simulink model "GVCU_HIL_simscape"  (R2026a)
settings: Solver=ode3  StartTime=0  StopTime=10  FixedStep=0.001
model workspace (MAT data in the model file):
  CANoelibParameters : object (value not decoded)
values from neighbouring files (symbols this model uses):
  acc_pedal_data = pedal_data.accelerator_pedal_position_t0    [Init_Simscape_main.m]
  acc_pedal_time = pedal_data.t0    [Init_Simscape_main.m]
  brk_pedal_data = brake_pedal_data.shared_brakes_drvrBrkPedlPerc_t0    [Init_Simscape_main.m]
  brk_pedal_time = brake_pedal_data.t0    [Init_Simscape_main.m]
  cycle_len = zeros(1, num_cycles)    [Init_Simscape_main.m]
  cycle_speed_matrix = zeros(max_cycle_len, num_cycles)    [Init_Simscape_main.m]
  cycle_time_matrix = zeros(max_cycle_len, num_cycles)    [Init_Simscape_main.m]
  veh_speed_data = speed_data.shared_dynamicsVso_vehVelLgt_t0    [Init_Simscape_main.m]
  veh_speed_time = speed_data.t0    [Init_Simscape_main.m]
undefined symbols (not defined in the file or in its folder): Active, aero, AuxActive, bat, brake, config, environment, FL, FL_prs_voltage, FR, FR_prs_voltage, front, pos, powertrain, rear, RL, RL_prs_voltage, RR, RR_prs_voltage, tir, veh, VGetRawValueFlag, Voltage, VT2816_1_Ch1, VT2816_1_Ch2, VT2816_1_Ch3, VT2816_1_Ch4, VT2816_3_Ch13, VT2816_3_Ch14, VT7101_1_Out2, VTS, X, Y, Z
libraries: sm_lib x358, fl_lib x272, nesl_utility x193, canoelib x127, sdl_lib x36, autolibsharedcoupling x21, autolibcoupling x9, slpidlib x7, simulink x3, autolibshareddiff x3, autolibshared x3, autolibutils x1
(part 4 of 17)

== system GVCU_HIL_simscape/GVCU - HiL/Message Output17 ==
  In1 : Inport
  Bus Selector : BusSelector  OutputSignals=available_charge_current,available_discharge_current,bms_state,dcdc_contactor,e2e_alive_counter_disabled,e2e_checksum_disabled,front_hv_bat_fan_req,front_hv_bat_pump_req,hv_on_req_lv_charging,hvac_contactor,obc_contactor
  S-Function_1 : S-Function  FunctionName=sigout  Parameters=dbName;nodeName;msgName;11;'available_charge_current';'available_discharge_current';'bms_state';'dcdc_contactor';'e2e_alive_counter_disabled';'e2e_checksum_disabled';'front_hv_bat_fan_req';'front_hv_bat_pump_req';'hv_on_req_lv_charging';'hvac_contactor';'obc_contactor';VGetRawValueFlag(rawValue);'inherited'  SFunctionDeploymentMode=off  EnableBusSupport=off
      settings: AttributesFormatString=available_charge_current\navailable_discharge_current\nbms_state\ndcdc_contactor\ne2e_alive_counter_disabled\ne2e_checksum_disabled\nfront_hv_bat_fan_req\nfront_hv_bat_pump_req\nhv_on_req_lv_charging\nhvac_contactor\nobc_contactor\n
  wires:
  In1/1 -> Bus Selector/1
  Bus Selector/1 -> S-Function_1/1  "<available_charge_current>"
  Bus Selector/2 -> S-Function_1/2  "<available_discharge_current>"
  Bus Selector/3 -> S-Function_1/3  "<bms_state>"
  Bus Selector/4 -> S-Function_1/4  "<dcdc_contactor>"
  Bus Selector/5 -> S-Function_1/5  "<e2e_alive_counter_disabled>"
  Bus Selector/6 -> S-Function_1/6  "<e2e_checksum_disabled>"
  Bus Selector/7 -> S-Function_1/7  "<front_hv_bat_fan_req>"
  Bus Selector/8 -> S-Function_1/8  "<front_hv_bat_pump_req>"
  Bus Selector/9 -> S-Function_1/9  "<hv_on_req_lv_charging>"
  Bus Selector/10 -> S-Function_1/10  "<hvac_contactor>"
  Bus Selector/11 -> S-Function_1/11  "<obc_contactor>"

== system GVCU_HIL_simscape/GVCU - HiL/Message Output18 ==
  In1 : Inport
  Bus Selector : BusSelector  OutputSignals=e2e_alive_counter_disabled,e2e_checksum_disabled,soc,soc_predictive,soc_predictive_v,soc_v,soe,soe_v,soh,soh_v,thermal_runaway_detection
  S-Function_1 : S-Function  FunctionName=sigout  Parameters=dbName;nodeName;msgName;11;'e2e_alive_counter_disabled';'e2e_checksum_disabled';'soc';'soc_predictive';'soc_predictive_v';'soc_v';'soe';'soe_v';'soh';'soh_v';'thermal_runaway_detection';VGetRawValueFlag(rawValue);'inherited'  SFunctionDeploymentMode=off  EnableBusSupport=off
      settings: AttributesFormatString=e2e_alive_counter_disabled\ne2e_checksum_disabled\nsoc\nsoc_predictive\nsoc_predictive_v\nsoc_v\nsoe\nsoe_v\nsoh\nsoh_v\nthermal_runaway_detection\n
  wires:
  In1/1 -> Bus Selector/1
  Bus Selector/10 -> S-Function_1/1, S-Function_1/10  "<soh_v>"
  Bus Selector/1 -> S-Function_1/2  "<e2e_alive_counter_disabled>"
  Bus Selector/2 -> S-Function_1/3  "<e2e_checksum_disabled>"
  Bus Selector/3 -> S-Function_1/4  "<soc>"
  Bus Selector/7 -> S-Function_1/5  "<soe>"
  Bus Selector/9 -> S-Function_1/6, S-Function_1/9  "<soh>"
  Bus Selector/11 -> S-Function_1/7, S-Function_1/11  "<thermal_runaway_detection>"
  Bus Selector/8 -> S-Function_1/8  "<soe_v>"

== system GVCU_HIL_simscape/GVCU - HiL/Message Output2 ==
  In1 : Inport
  Bus Selector : BusSelector  OutputSignals=third_shaft_speed,third_shaft_speed_v
  S-Function_1 : S-Function  FunctionName=sigout  Parameters=dbName;nodeName;msgName;2;'third_shaft_speed';'third_shaft_speed_v';VGetRawValueFlag(rawValue);'inherited'  SFunctionDeploymentMode=off  EnableBusSupport=off
      settings: AttributesFormatString=third_shaft_speed\nthird_shaft_speed_v\n
  wires:
  In1/1 -> Bus Selector/1
  Bus Selector/1 -> S-Function_1/1  "<third_shaft_speed>"
  Bus Selector/2 -> S-Function_1/2  "<third_shaft_speed_v>"

== system GVCU_HIL_simscape/GVCU - HiL/Message Output21 ==
  In1 : Inport
  Bus Selector : BusSelector  OutputSignals=active_mode,brake_pedal_applied,brake_pedal_travel_mm,brake_pedal_travel_mm_v,brake_pedal_travel_perc,brake_pedal_travel_perc_v,brake_pedal_travel_sensor_sts,e2e_alive_counter,e2e_checksum,position_motor,position_motor_v
  S-Function_1 : S-Function  FunctionName=sigout  Parameters=dbName;nodeName;msgName;11;'active_mode';'brake_pedal_applied';'brake_pedal_travel_mm';'brake_pedal_travel_mm_v';'brake_pedal_travel_perc';'brake_pedal_travel_perc_v';'brake_pedal_travel_sensor_sts';'e2e_alive_counter';'e2e_checksum';'position_motor';'position_motor_v';VGetRawValueFlag(rawValue);'inherited'  SFunctionDeploymentMode=off  EnableBusSupport=off
      settings: AttributesFormatString=active_mode\nbrake_pedal_applied\nbrake_pedal_travel_mm\nbrake_pedal_travel_mm_v\nbrake_pedal_travel_perc\nbrake_pedal_travel_perc_v\nbrake_pedal_travel_sensor_sts\ne2e_alive_counter\ne2e_checksum\nposition_motor\nposition_motor_v\n
  wires:
  In1/1 -> Bus Selector/1
  Bus Selector/7 -> S-Function_1/1  "<brake_pedal_travel_sensor_sts>"
  Bus Selector/1 -> S-Function_1/2  "<active_mode>"
  Bus Selector/4 -> S-Function_1/3  "<brake_pedal_travel_mm_v>"
  Bus Selector/8 -> S-Function_1/4  "<e2e_alive_counter>"
  Bus Selector/9 -> S-Function_1/5  "<e2e_checksum>"
  Bus Selector/11 -> S-Function_1/6, S-Function_1/11  "<position_motor_v>"
  Bus Selector/6 -> S-Function_1/7  "<brake_pedal_travel_perc_v>"
  Bus Selector/2 -> S-Function_1/8  "<brake_pedal_applied>"
  Bus Selector/10 -> S-Function_1/9  "<position_motor>"
  Bus Selector/3 -> S-Function_1/10  "<brake_pedal_travel_mm>"

== system GVCU_HIL_simscape/GVCU - HiL/Message Output3 ==
  In1 : Inport
  Bus Selector : BusSelector  OutputSignals=auto_shift_perf_mod_swt_req,ddc_perf_mod_swt_req,e2e_alive_counter_disabled,e2e_checksum_disabled,eps_perf_mod_swt_req,pedl_map_perf_mod_swt_req,perf_mod_swt_req,perf_stgy_perf_mod_swt_req,rgn_perf_mod_swt_req,rhc_perf_mod_swt_req
  S-Function_1 : S-Function  FunctionName=sigout  Parameters=dbName;nodeName;msgName;10;'auto_shift_perf_mod_swt_req';'ddc_perf_mod_swt_req';'e2e_alive_counter_disabled';'e2e_checksum_disabled';'eps_perf_mod_swt_req';'pedl_map_perf_mod_swt_req';'perf_mod_swt_req';'perf_stgy_perf_mod_swt_req';'rgn_perf_mod_swt_req';'rhc_perf_mod_swt_req';VGetRawValueFlag(rawValue);'inherited'  SFunctionDeploymentMode=off  EnableBusSupport=off
      settings: AttributesFormatString=auto_shift_perf_mod_swt_req\nddc_perf_mod_swt_req\ne2e_alive_counter_disabled\ne2e_checksum_disabled\neps_perf_mod_swt_req\npedl_map_perf_mod_swt_req\nperf_mod_swt_req\nperf_stgy_perf_mod_swt_req\nrgn_perf_mod_swt_req\nrhc_perf_mod_swt_req\n
  wires:
  In1/1 -> Bus Selector/1
  Bus Selector/1 -> S-Function_1/1  "<auto_shift_perf_mod_swt_req>"
  Bus Selector/2 -> S-Function_1/2  "<ddc_perf_mod_swt_req>"
  ? -> S-Function_1/3  "<drift_mod_swt_req>"
  Bus Selector/3 -> S-Function_1/4  "<e2e_alive_counter_disabled>"
  Bus Selector/4 -> S-Function_1/5  "<e2e_checksum_disabled>"
  Bus Selector/5 -> S-Function_1/6  "<eps_perf_mod_swt_req>"
  Bus Selector/6 -> S-Function_1/7  "<pedl_map_perf_mod_swt_req>"
  Bus Selector/7 -> S-Function_1/8  "<perf_mod_swt_req>"
  Bus Selector/8 -> S-Function_1/9  "<perf_stgy_perf_mod_swt_req>"
  Bus Selector/9 -> S-Function_1/10  "<rgn_perf_mod_swt_req>"

== system GVCU_HIL_simscape/GVCU - HiL/Message Output7 ==
  In1 : Inport
  Bus Selector : BusSelector  OutputSignals=dtc_list_12v,dtc_list_48v,e2e_alive_counter_disabled,e2e_checksum_disabled,in_current_hv,in_voltage_hv,state_12v,state_48v,swt_ena_fb_12v,swt_ena_fb_48v
  S-Function_1 : S-Function  FunctionName=sigout  Parameters=dbName;nodeName;msgName;10;'dtc_list_12v';'dtc_list_48v';'e2e_alive_counter_disabled';'e2e_checksum_disabled';'in_current_hv';'in_voltage_hv';'state_12v';'state_48v';'swt_ena_fb_12v';'swt_ena_fb_48v';VGetRawValueFlag(rawValue);'inherited'  SFunctionDeploymentMode=off  EnableBusSupport=off
      settings: AttributesFormatString=dtc_list_12v\ndtc_list_48v\ne2e_alive_counter_disabled\ne2e_checksum_disabled\nin_current_hv\nin_voltage_hv\nstate_12v\nstate_48v\nswt_ena_fb_12v\nswt_ena_fb_48v\n
  wires:
  In1/1 -> Bus Selector/1
  Bus Selector/1 -> S-Function_1/1  "<dtc_list_12v>"
  Bus Selector/2 -> S-Function_1/2  "<dtc_list_48v>"
  Bus Selector/3 -> S-Function_1/3  "<e2e_alive_counter_disabled>"
  Bus Selector/4 -> S-Function_1/4  "<e2e_checksum_disabled>"
  Bus Selector/5 -> S-Function_1/5  "<in_current_hv>"
  Bus Selector/6 -> S-Function_1/6  "<in_voltage_hv>"
  Bus Selector/7 -> S-Function_1/7  "<state_12v>"
  Bus Selector/8 -> S-Function_1/8  "<state_48v>"
  Bus Selector/9 -> S-Function_1/9  "<swt_ena_fb_12v>"
  Bus Selector/10 -> S-Function_1/10  "<swt_ena_fb_48v>"

== system GVCU_HIL_simscape/GVCU - HiL/Message Output8 ==
  In1 : Inport
  Bus Selector : BusSelector  OutputSignals=available_power_12v,available_power_48v,current_output_12v,current_output_48v,dcdc_fan_req,dcdc_pump_req,e2e_alive_counter_disabled,e2e_checksum_disabled
  S-Function_1 : S-Function  FunctionName=sigout  Parameters=dbName;nodeName;msgName;8;'available_power_12v';'available_power_48v';'current_output_12v';'current_output_48v';'dcdc_fan_req';'dcdc_pump_req';'e2e_alive_counter_disabled';'e2e_checksum_disabled';VGetRawValueFlag(rawValue);'inherited'  SFunctionDeploymentMode=off  EnableBusSupport=off
      settings: AttributesFormatString=available_power_12v\navailable_power_48v\ncurrent_output_12v\ncurrent_output_48v\ndcdc_fan_req\ndcdc_pump_req\ne2e_alive_counter_disabled\ne2e_checksum_disabled\n
  wires:
  In1/1 -> Bus Selector/1
  Bus Selector/1 -> S-Function_1/1  "<available_power_12v>"
  Bus Selector/2 -> S-Function_1/2  "<available_power_48v>"
  Bus Selector/3 -> S-Function_1/3  "<current_output_12v>"
  Bus Selector/4 -> S-Function_1/4  "<current_output_48v>"
  Bus Selector/5 -> S-Function_1/5  "<dcdc_fan_req>"
  Bus Selector/6 -> S-Function_1/6  "<dcdc_pump_req>"
  Bus Selector/7 -> S-Function_1/7  "<e2e_alive_counter_disabled>"
  Bus Selector/8 -> S-Function_1/8  "<e2e_checksum_disabled>"

== system GVCU_HIL_simscape/Inverter/Message Output ==
  In1 : Inport
  Bus Selector : BusSelector  OutputSignals=ctrl_mode_feedback,dc_current,dc_voltage,e2e_alive_counter_disabled,e2e_checksum_disabled,fault_level,inv_enable_feedback,motor_enable_feedback,safe_state_method,safe_state_req_feedback,state_machine,torque_limit_reason
  S-Function_1 : S-Function  FunctionName=sigout  Parameters=dbName;nodeName;msgName;12;'ctrl_mode_feedback';'dc_current';'dc_voltage';'e2e_alive_counter_disabled';'e2e_checksum_disabled';'fault_level';'inv_enable_feedback';'motor_enable_feedback';'safe_state_method';'safe_state_req_feedback';'state_machine';'torque_limit_reason';VGetRawValueFlag(rawValue);'inherited'  SFunctionDeploymentMode=off  EnableBusSupport=off
      settings: AttributesFormatString=ctrl_mode_feedback\ndc_current\ndc_voltage\ne2e_alive_counter_disabled\ne2e_checksum_disabled\nfault_level\ninv_enable_feedback\nmotor_enable_feedback\nsafe_state_method\nsafe_state_req_feedback\nstate_machine\ntorque_limit_reason\n
  wires:
  In1/1 -> Bus Selector/1
  Bus Selector/1 -> S-Function_1/1  "<ctrl_mode_feedback>"
  Bus Selector/2 -> S-Function_1/2  "<dc_current>"
  Bus Selector/3 -> S-Function_1/3  "<dc_voltage>"
  Bus Selector/4 -> S-Function_1/4  "<e2e_alive_counter_disabled>"
  Bus Selector/5 -> S-Function_1/5  "<e2e_checksum_disabled>"
  Bus Selector/6 -> S-Function_1/6  "<fault_level>"
  Bus Selector/7 -> S-Function_1/7  "<inv_enable_feedback>"
  Bus Selector/8 -> S-Function_1/8  "<motor_enable_feedback>"
  Bus Selector/9 -> S-Function_1/9  "<safe_state_method>"
  Bus Selector/10 -> S-Function_1/10  "<safe_state_req_feedback>"
  Bus Selector/11 -> S-Function_1/11  "<state_machine>"
  Bus Selector/12 -> S-Function_1/12  "<torque_limit_reason>"

== system GVCU_HIL_simscape/Inverter/Message Output1 ==
  In1 : Inport
  Bus Selector : BusSelector  OutputSignals=e2e_alive_counter_disabled,e2e_checksum_disabled,motor_speed,motor_speed_valid_bit,pos_offset_a,pos_offset_b
  S-Function_1 : S-Function  FunctionName=sigout  Parameters=dbName;nodeName;msgName;6;'e2e_alive_counter_disabled';'e2e_checksum_disabled';'motor_speed';'motor_speed_valid_bit';'pos_offset_a';'pos_offset_b';VGetRawValueFlag(rawValue);'inherited'  SFunctionDeploymentMode=off  EnableBusSupport=off
      settings: AttributesFormatString=e2e_alive_counter_disabled\ne2e_checksum_disabled\nmotor_speed\nmotor_speed_valid_bit\npos_offset_a\npos_offset_b\n
  wires:
  In1/1 -> Bus Selector/1
  Bus Selector/1 -> S-Function_1/1  "<e2e_alive_counter_disabled>"
  Bus Selector/2 -> S-Function_1/2  "<e2e_checksum_disabled>"
  Bus Selector/3 -> S-Function_1/3  "<motor_speed>"
  Bus Selector/4 -> S-Function_1/4  "<motor_speed_valid_bit>"
  Bus Selector/5 -> S-Function_1/5  "<pos_offset_a>"
  Bus Selector/6 -> S-Function_1/6  "<pos_offset_b>"

== system GVCU_HIL_simscape/Inverter/Message Output2 ==
  In1 : Inport
  Bus Selector : BusSelector  OutputSignals=can_comm_loss_error,can_comm_loss_warning,can_e2e,coolant_t_fault,coolant_t_rationality,coolant_t_sensing,coolant_t_warning,crash_signal,dc_link_t_fault,dc_link_t_rationality,dc_link_t_sensing,dc_link_t_warning,driver_t_fault,driver_t_rationality,driver_t_sensing,driver_t_warning,e2e_alive_counter_disabled,e2e_checksum_disabled,gate_driver_bist_fault,gate_driver_fault,gate_driver_warning,inverter_boards_t_fault,inverter_boards_t_rationality,inverter_boards_t_sensing,inverter_boards_t_warning,ipc_lock_cm,ipc_lock_main,lv_ext_supply_ov,lv_ext_supply_uv,lv_int_supply,lv_self_check_main,mcu_bist_fault,mcu_fault,mosfet_t_fault,mosfet_t_imbalance,mosfet_t_rationality,mosfet_t_sensing,mosfet_t_warning,motor_t_fault,motor_t_rationality,motor_t_sensing,motor_t_warning,sbc_bist_fault,sbc_fault,sw_compatibility,task_alive_cm,task_alive_main,task_deadline_cm,task_deadline_main,y_cap_ctrl_u
  S-Function_1 : S-Function  FunctionName=sigout  Parameters=dbName;nodeName;msgName;50;'can_comm_loss_error';'can_comm_loss_warning';'can_e2e';'coolant_t_fault';'coolant_t_rationality';'coolant_t_sensing';'coolant_t_warning';'crash_signal';'dc_link_t_fault';'dc_link_t_rationality';'dc_link_t_sensing';'dc_link_t_warning';'driver_t_fault';'driver_t_rationality';'driver_t_sensing';'driver_t_warning';'e2e_alive_counter_disabled';'e2e_checksum_disabled';'gate_driver_bist_fault';'gate_driver_fault';'gate_driver_warning';'inverter_boards_t_fault';'inverter_boards_t_rationality';'inverter_boards_t_sensing';'inverter_boards_t_warning';'ipc_lock_cm';'ipc_lock_main';'lv_ext_supply_ov';'lv_ext_supply_uv';'lv_int_supply';'lv_self_check_main';'mcu_bist_fault';'mcu_fault';'mosfet_t_fault';'mosfet_t_imbalance';'mosfet_t_rationality';'mosfet_t_sensing';'mosfet_t_warning';'motor_t_fault';'motor_t_rationality';'motor_t_sensing';'motor_t_warning';'sbc_bist_fault';'sbc_fault';'sw_compatibility';'task_alive_cm';'task_alive_main';'task_deadline_cm';'task_deadline_main';'y_cap_ctrl_u';VGetRawValueFlag(rawValue);'inherited'  SFunctionDeploymentMode=off  EnableBusSupport=off
      settings: AttributesFormatString=can_comm_loss_error\ncan_comm_loss_warning\ncan_e2e\ncoolant_t_fault\ncoolant_t_rationality\ncoolant_t_sensing\ncoolant_t_warning\ncrash_signal\ndc_link_t_fault\ndc_link_t_rationality\ndc_link_t_sensing\ndc_link_t_warning\ndriver_t_fault\ndriver_t_rationality\ndriver_t_sensing\ndriver_t_warning\ne2e_alive_counter_disabled\ne2e_checksum_disabled\ngate_driver_bist_fault\ngate_driver_fault\ngate_driver_warning\ninverter_boards_t_fault\ninverter_boards_t_rationality\ninverter_boards_t_sensing\ninverter_boards_t_warning\nipc_lock_cm\nipc_lock_main\nlv_ext_supply_ov\nlv_ext_supply_uv\nlv_int_supply\nlv_self_check_main\nmcu_bist_fault\nmcu_fault\nmosfet_t_fault\nmosfet_t_imbalance\nmosfet_t_rationality\nmosfet_t_sensing\nmosfet_t_warning\nmotor_t_fault\nmotor_t_rationality\nmotor_t_sensing\nmotor_t_warning\nsbc_bist_fault\nsbc_fault\nsw_compatibility\ntask_alive_cm\ntask_alive_main\ntask_deadline_cm\ntask_deadline_main\ny_cap_ctrl_u\n
  wires:
  In1/1 -> Bus Selector/1
  Bus Selector/1 -> S-Function_1/1  "<can_comm_loss_error>"
  Bus Selector/2 -> S-Function_1/2  "<can_comm_loss_warning>"
  Bus Selector/3 -> S-Function_1/3  "<can_e2e>"
  Bus Selector/4 -> S-Function_1/4  "<coolant_t_fault>"
  Bus Selector/5 -> S-Function_1/5  "<coolant_t_rationality>"
  Bus Selector/6 -> S-Function_1/6  "<coolant_t_sensing>"
  Bus Selector/7 -> S-Function_1/7  "<coolant_t_warning>"
  Bus Selector/8 -> S-Function_1/8  "<crash_signal>"
  Bus Selector/9 -> S-Function_1/9  "<dc_link_t_fault>"
  Bus Selector/10 -> S-Function_1/10  "<dc_link_t_rationality>"
  Bus Selector/11 -> S-Function_1/11  "<dc_link_t_sensing>"
  Bus Selector/12 -> S-Function_1/12  "<dc_link_t_warning>"
  Bus Selector/13 -> S-Function_1/13  "<driver_t_fault>"
  Bus Selector/14 -> S-Function_1/14  "<driver_t_rationality>"
  Bus Selector/15 -> S-Function_1/15  "<driver_t_sensing>"
  Bus Selector/16 -> S-Function_1/16  "<driver_t_warning>"
  Bus Selector/17 -> S-Function_1/17  "<e2e_alive_counter_disabled>"
  Bus Selector/18 -> S-Function_1/18  "<e2e_checksum_disabled>"
  Bus Selector/19 -> S-Function_1/19  "<gate_driver_bist_fault>"
  Bus Selector/20 -> S-Function_1/20  "<gate_driver_fault>"
  Bus Selector/21 -> S-Function_1/21  "<gate_driver_warning>"
  Bus Selector/22 -> S-Function_1/22  "<inverter_boards_t_fault>"
  Bus Selector/23 -> S-Function_1/23  "<inverter_boards_t_rationality>"
  Bus Selector/24 -> S-Function_1/24  "<inverter_boards_t_sensing>"
  Bus Selector/25 -> S-Function_1/25  "<inverter_boards_t_warning>"
  Bus Selector/26 -> S-Function_1/26  "<ipc_lock_cm>"
  Bus Selector/27 -> S-Function_1/27  "<ipc_lock_main>"
  Bus Selector/28 -> S-Function_1/28  "<lv_ext_supply_ov>"
  Bus Selector/29 -> S-Function_1/29  "<lv_ext_supply_uv>"
  Bus Selector/30 -> S-Function_1/30  "<lv_int_supply>"
  Bus Selector/31 -> S-Function_1/31  "<lv_self_check_main>"
  Bus Selector/32 -> S-Function_1/32  "<mcu_bist_fault>"
  Bus Selector/33 -> S-Function_1/33  "<mcu_fault>"
  Bus Selector/34 -> S-Function_1/34  "<mosfet_t_fault>"
  Bus Selector/36 -> S-Function_1/35  "<mosfet_t_rationality>"
  Bus Selector/37 -> S-Function_1/36  "<mosfet_t_sensing>"
  Bus Selector/38 -> S-Function_1/37  "<mosfet_t_warning>"
  Bus Selector/39 -> S-Function_1/38  "<motor_t_fault>"
  Bus Selector/40 -> S-Function_1/39  "<motor_t_rationality>"
  Bus Selector/41 -> S-Function_1/40  "<motor_t_sensing>"
  Bus Selector/42 -> S-Function_1/41  "<motor_t_warning>"
  Bus Selector/43 -> S-Function_1/42  "<sbc_bist_fault>"
  Bus Selector/44 -> S-Function_1/43  "<sbc_fault>"
  Bus Selector/45 -> S-Function_1/44  "<sw_compatibility>"
  Bus Selector/46 -> S-Function_1/45  "<task_alive_cm>"
  Bus Selector/47 -> S-Function_1/46  "<task_alive_main>"
  Bus Selector/48 -> S-Function_1/47  "<task_deadline_cm>"
  Bus Selector/49 -> S-Function_1/48  "<task_deadline_main>"
  Bus Selector/50 -> S-Function_1/49, S-Function_1/50  "<y_cap_ctrl_u>"

== system GVCU_HIL_simscape/Inverter/Message Output3 ==
  In1 : Inport
  Bus Selector : BusSelector  OutputSignals=coolant_temp,dc_cap_temp_1,dc_cap_temp_2,driver_board_temp_max,e2e_alive_counter_disabled,e2e_checksum_disabled,mosfet_temp_max,pcb_temp
  S-Function_1 : S-Function  FunctionName=sigout  Parameters=dbName;nodeName;msgName;8;'coolant_temp';'dc_cap_temp_1';'dc_cap_temp_2';'driver_board_temp_max';'e2e_alive_counter_disabled';'e2e_checksum_disabled';'mosfet_temp_max';'pcb_temp';VGetRawValueFlag(rawValue);'inherited'  SFunctionDeploymentMode=off  EnableBusSupport=off
      settings: AttributesFormatString=coolant_temp\ndc_cap_temp_1\ndc_cap_temp_2\ndriver_board_temp_max\ne2e_alive_counter_disabled\ne2e_checksum_disabled\nmosfet_temp_max\npcb_temp\n
  wires:
  In1/1 -> Bus Selector/1
  Bus Selector/1 -> S-Function_1/1  "<coolant_temp>"
  Bus Selector/2 -> S-Function_1/2  "<dc_cap_temp_1>"
  Bus Selector/3 -> S-Function_1/3  "<dc_cap_temp_2>"
  Bus Selector/4 -> S-Function_1/4  "<driver_board_temp_max>"
  Bus Selector/5 -> S-Function_1/5  "<e2e_alive_counter_disabled>"
  Bus Selector/6 -> S-Function_1/6  "<e2e_checksum_disabled>"
  Bus Selector/7 -> S-Function_1/7  "<mosfet_temp_max>"
  Bus Selector/8 -> S-Function_1/8  "<pcb_temp>"

== system GVCU_HIL_simscape/Inverter/Message Output4 ==
  In1 : Inport
  Bus Selector : BusSelector  OutputSignals=e2e_alive_counter_disabled,e2e_checksum_disabled,motor_temp_a1,motor_temp_a2,motor_temp_a3,motor_temp_a4
  S-Function_1 : S-Function  FunctionName=sigout  Parameters=dbName;nodeName;msgName;6;'e2e_alive_counter_disabled';'e2e_checksum_disabled';'motor_temp_a1';'motor_temp_a2';'motor_temp_a3';'motor_temp_a4';VGetRawValueFlag(rawValue);'inherited'  SFunctionDeploymentMode=off  EnableBusSupport=off
      settings: AttributesFormatString=e2e_alive_counter_disabled\ne2e_checksum_disabled\nmotor_temp_a1\nmotor_temp_a2\nmotor_temp_a3\nmotor_temp_a4\n
  wires:
  In1/1 -> Bus Selector/1
  Bus Selector/1 -> S-Function_1/1  "<e2e_alive_counter_disabled>"
  Bus Selector/2 -> S-Function_1/2  "<e2e_checksum_disabled>"
  Bus Selector/3 -> S-Function_1/3  "<motor_temp_a1>"
  Bus Selector/4 -> S-Function_1/4  "<motor_temp_a2>"
  Bus Selector/5 -> S-Function_1/5  "<motor_temp_a3>"
  Bus Selector/6 -> S-Function_1/6  "<motor_temp_a4>"

== system GVCU_HIL_simscape/Inverter/Message Output5 ==
  In1 : Inport
  Bus Selector : BusSelector  OutputSignals=actual_torque,available_torque_neg,available_torque_pos,e2e_alive_counter_disabled,e2e_checksum_disabled,requested_torque
  S-Function_1 : S-Function  FunctionName=sigout  Parameters=dbName;nodeName;msgName;6;'actual_torque';'available_torque_neg';'available_torque_pos';'e2e_alive_counter_disabled';'e2e_checksum_disabled';'requested_torque';VGetRawValueFlag(rawValue);'inherited'  SFunctionDeploymentMode=off  EnableBusSupport=off
      settings: AttributesFormatString=actual_torque\navailable_torque_neg\navailable_torque_pos\ne2e_alive_counter_disabled\ne2e_checksum_disabled\nrequested_torque\n
  wires:
  In1/1 -> Bus Selector/1
  Bus Selector/1 -> S-Function_1/1  "<actual_torque>"
  Bus Selector/2 -> S-Function_1/2  "<available_torque_neg>"
  Bus Selector/3 -> S-Function_1/3  "<available_torque_pos>"
  Bus Selector/4 -> S-Function_1/4  "<e2e_alive_counter_disabled>"
  Bus Selector/5 -> S-Function_1/5  "<e2e_checksum_disabled>"
  Bus Selector/6 -> S-Function_1/6  "<requested_torque>"

== system GVCU_HIL_simscape/Inverter/Message Output6 ==
  In1 : Inport
  Bus Selector : BusSelector  OutputSignals=ac_i_sensor_calibration,ac_i_sensor_oor,ac_phase_i_imbalance,ac_phase_i_oc,ac_phase_loss,ac_phase_short,ac_phase_u_rationnality,ctrl_mode_rationnality,dc_bus_i_oc,dc_bus_i_rationnality,dc_bus_i_sensing,dc_bus_u_ov,dc_bus_u_rationnality,dc_bus_u_sensing,dc_bus_u_uv,e2e_alive_counter_disabled,e2e_checksum_disabled,hv_self_check_ctrl,ipc_lock_ctrl,lv_self_check_ctrl,motor_over_speed,motor_speed_rationnality,motor_stall,rslv_bist_fault,rslv_fault,rslv_offset,task_alive_ctrl,task_deadline_ctrl,trq_command_rationnality,trq_estimation_rationnality
  S-Function_1 : S-Function  FunctionName=sigout  Parameters=dbName;nodeName;msgName;30;'ac_i_sensor_calibration';'ac_i_sensor_oor';'ac_phase_i_imbalance';'ac_phase_i_oc';'ac_phase_loss';'ac_phase_short';'ac_phase_u_rationnality';'ctrl_mode_rationnality';'dc_bus_i_oc';'dc_bus_i_rationnality';'dc_bus_i_sensing';'dc_bus_u_ov';'dc_bus_u_rationnality';'dc_bus_u_sensing';'dc_bus_u_uv';'e2e_alive_counter_disabled';'e2e_checksum_disabled';'hv_self_check_ctrl';'ipc_lock_ctrl';'lv_self_check_ctrl';'motor_over_speed';'motor_speed_rationnality';'motor_stall';'rslv_bist_fault';'rslv_fault';'rslv_offset';'task_alive_ctrl';'task_deadline_ctrl';'trq_command_rationnality';'trq_estimation_rationnality';VGetRawValueFlag(rawValue);'inherited'  SFunctionDeploymentMode=off  EnableBusSupport=off
      settings: AttributesFormatString=ac_i_sensor_calibration\nac_i_sensor_oor\nac_phase_i_imbalance\nac_phase_i_oc\nac_phase_loss\nac_phase_short\nac_phase_u_rationnality\nctrl_mode_rationnality\ndc_bus_i_oc\ndc_bus_i_rationnality\ndc_bus_i_sensing\ndc_bus_u_ov\ndc_bus_u_rationnality\ndc_bus_u_sensing\ndc_bus_u_uv\ne2e_alive_counter_disabled\ne2e_checksum_disabled\nhv_self_check_ctrl\nipc_lock_ctrl\nlv_self_check_ctrl\nmotor_over_speed\nmotor_speed_rationnality\nmotor_stall\nrslv_bist_fault\nrslv_fault\nrslv_offset\ntask_alive_ctrl\ntask_deadline_ctrl\ntrq_command_rationnality\ntrq_estimation_rationnality\n
  wires:
  In1/1 -> Bus Selector/1
  Bus Selector/1 -> S-Function_1/1  "<ac_i_sensor_calibration>"
  Bus Selector/2 -> S-Function_1/2  "<ac_i_sensor_oor>"
  Bus Selector/3 -> S-Function_1/3  "<ac_phase_i_imbalance>"
  Bus Selector/4 -> S-Function_1/4  "<ac_phase_i_oc>"
  Bus Selector/5 -> S-Function_1/5  "<ac_phase_loss>"
  Bus Selector/6 -> S-Function_1/6  "<ac_phase_short>"
  Bus Selector/7 -> S-Function_1/7  "<ac_phase_u_rationnality>"
  Bus Selector/8 -> S-Function_1/8  "<ctrl_mode_rationnality>"
  Bus Selector/9 -> S-Function_1/9  "<dc_bus_i_oc>"
  Bus Selector/10 -> S-Function_1/10  "<dc_bus_i_rationnality>"
  Bus Selector/11 -> S-Function_1/11  "<dc_bus_i_sensing>"
  Bus Selector/12 -> S-Function_1/12  "<dc_bus_u_ov>"
  Bus Selector/13 -> S-Function_1/13  "<dc_bus_u_rationnality>"
  Bus Selector/14 -> S-Function_1/14  "<dc_bus_u_sensing>"
  Bus Selector/15 -> S-Function_1/15  "<dc_bus_u_uv>"
  Bus Selector/16 -> S-Function_1/16  "<e2e_alive_counter_disabled>"
  Bus Selector/17 -> S-Function_1/17  "<e2e_checksum_disabled>"
  Bus Selector/18 -> S-Function_1/18  "<hv_self_check_ctrl>"
  Bus Selector/19 -> S-Function_1/19  "<ipc_lock_ctrl>"
  Bus Selector/20 -> S-Function_1/20  "<lv_self_check_ctrl>"
  Bus Selector/21 -> S-Function_1/21  "<motor_over_speed>"
  Bus Selector/22 -> S-Function_1/22  "<motor_speed_rationnality>"
  Bus Selector/23 -> S-Function_1/23  "<motor_stall>"
  Bus Selector/24 -> S-Function_1/24  "<rslv_bist_fault>"
  Bus Selector/25 -> S-Function_1/25  "<rslv_fault>"
  Bus Selector/26 -> S-Function_1/26  "<rslv_offset>"
  Bus Selector/27 -> S-Function_1/27  "<task_alive_ctrl>"
  Bus Selector/28 -> S-Function_1/28  "<task_deadline_ctrl>"
  Bus Selector/29 -> S-Function_1/29  "<trq_command_rationnality>"
  Bus Selector/30 -> S-Function_1/30  "<trq_estimation_rationnality>"

== system GVCU_HIL_simscape/Inverter/Message Output7 ==
  In1 : Inport
  Bus Selector : BusSelector  OutputSignals=e2e_alive_counter_disabled,e2e_checksum_disabled,mechanical_pwr_out
  S-Function_1 : S-Function  FunctionName=sigout  Parameters=dbName;nodeName;msgName;3;'e2e_alive_counter_disabled';'e2e_checksum_disabled';'mechanical_pwr_out';VGetRawValueFlag(rawValue);'inherited'  SFunctionDeploymentMode=off  EnableBusSupport=off
      settings: AttributesFormatString=e2e_alive_counter_disabled\ne2e_checksum_disabled\nmechanical_pwr_out\n
  wires:
  Bus Selector/3 -> S-Function_1/3  "<mechanical_pwr_out>"
  Bus Selector/2 -> S-Function_1/2  "<e2e_checksum_disabled>"
  Bus Selector/1 -> S-Function_1/1  "<e2e_alive_counter_disabled>"
  In1/1 -> Bus Selector/1

== system GVCU_HIL_simscape/Powertrain (EV)/AWD_Powertrain1 ==
  DM_Trq : Inport
  Veh : Inport  Port=2
  Central axle : Subsystem
  Front Axle : Subsystem
  Goto : Goto  Commented=on  GotoTag=Front_axle_sen  TagVisibility=global
  Mux : Mux
  Rear Axle : Subsystem
  Terminator1 : Terminator
  Transfer Case : autolibshareddiff/Transfer Case  DiffEffModelPopup=Constant  InterpMethod=Linear point-slope  extTamb=off  TrqSplitRatioMode=off  SpdLockMode=off  shaftSwitchMask=To the left of center-line  Ndiff=1  Jd=.1  bd=1e-3  Jw1=.1  bw1=1e-3  Jw2=.1  bw2=1e-3  omegaw1o=0  omegaw2o=0  eta=1  eta_tbl=reshape([0.64 0.76 0.8 0.81 0.83 0.84 0.84 0.56 0.73 0.78 0.8 0.83 0.84 0.84 0.54 0.71 0.77 0.8 0.82 0.84 0.84 0.53 0.71 0.77 0.8 0.83 0.84 0.84 0.51 0.71 0.77 0.8 0.83 0.84 0.85 0.52 0.7 0.77 0.8 0.83 0.84 0.85 0.51 0.71 0.76 0.79 0.83 0.84 0.85 0.5 0.69 0.76 0.79 0.82 0.84 0.85 0.45 0.68 0.75 0.78 0.82 0.84 0.85 0.43 0.67 0.74 0.78 0.81 0.83 0.84 0.38 0.63 0.71 0.75 0.8 0.82 0.83 0.81 0.86 0.88 0.89 0.89 0.89 0.9 0.77 0.85 0.87 0.88 0.89 0.9 0.9 0.72 0.82 0.86 0.87 0.88 0.89 0.9 0.68 0.8 0.84 0.86 0.88 0.89 0.89 0.67 0.8 0.84 0.86 0.88 0.89 0.9 0.67 0.8 0.84 0.86 0.88 0.89 0.9 0.65 0.8 0.84 0.86 0.88 0.89 0.9 0.64 0.79 0.83 0.86 0.88 0.89 0.9 0.63 0.78 0.83 0.86 0.88 0.89 0.9 0.59 0.76 0.82 0.85 0.87 0.89 0.9 0.53 0.73 0.8 0.83 0.86 0.88 0.89], 7, 11, 2)  Trq_bpts=[25, 50, 75, 100, 150, 200, 250]  omega_bpts=[52.4 78.5 105 131 157 183 209 262 314 419 524]  Temp_bpts=[290 358]  Tamb=297.15  maxAbsSpd=5e3  aMode=1  TrqSplitRatio=0.5  SpdLock=0
      settings: LibrarySourceBlock=autolibdiff/Transfer Case
  Transfer Case1 : autolibshareddiff/Transfer Case  Commented=on  DiffEffModelPopup=Constant  InterpMethod=Linear point-slope  extTamb=off  TrqSplitRatioMode=off  SpdLockMode=off  shaftSwitchMask=To the left of center-line  Ndiff=1  Jd=.1  bd=1e-3  Jw1=.1  bw1=1e-3  Jw2=.1  bw2=1e-3  omegaw1o=0  omegaw2o=0  eta=1  eta_tbl=reshape([0.64 0.76 0.8 0.81 0.83 0.84 0.84 0.56 0.73 0.78 0.8 0.83 0.84 0.84 0.54 0.71 0.77 0.8 0.82 0.84 0.84 0.53 0.71 0.77 0.8 0.83 0.84 0.84 0.51 0.71 0.77 0.8 0.83 0.84 0.85 0.52 0.7 0.77 0.8 0.83 0.84 0.85 0.51 0.71 0.76 0.79 0.83 0.84 0.85 0.5 0.69 0.76 0.79 0.82 0.84 0.85 0.45 0.68 0.75 0.78 0.82 0.84 0.85 0.43 0.67 0.74 0.78 0.81 0.83 0.84 0.38 0.63 0.71 0.75 0.8 0.82 0.83 0.81 0.86 0.88 0.89 0.89 0.89 0.9 0.77 0.85 0.87 0.88 0.89 0.9 0.9 0.72 0.82 0.86 0.87 0.88 0.89 0.9 0.68 0.8 0.84 0.86 0.88 0.89 0.89 0.67 0.8 0.84 0.86 0.88 0.89 0.9 0.67 0.8 0.84 0.86 0.88 0.89 0.9 0.65 0.8 0.84 0.86 0.88 0.89 0.9 0.64 0.79 0.83 0.86 0.88 0.89 0.9 0.63 0.78 0.83 0.86 0.88 0.89 0.9 0.59 0.76 0.82 0.85 0.87 0.89 0.9 0.53 0.73 0.8 0.83 0.86 0.88 0.89], 7, 11, 2)  Trq_bpts=[25, 50, 75, 100, 150, 200, 250]  omega_bpts=[52.4 78.5 105 131 157 183 209 262 314 419 524]  Temp_bpts=[290 358]  Tamb=297.15  maxAbsSpd=5e3  aMode=1  TrqSplitRatio=0.5  SpdLock=0
      settings: LibrarySourceBlock=autolibdiff/Transfer Case
  omega_to_freq_central : Gain  Commented=on  Gain=38/(2*pi)
  DM_Spd : Outport
  Axl_Trq : Outport  Port=2
  tag scope: Axl_centre_Spd=global
  wires:
  Mux/1 -> Axl_Trq/1
  Transfer Case/2 -> DM_Spd/1
  DM_Trq/1 -> Transfer Case/1
  Rear Axle/1(Trq_RL) -> Mux/3  "T_RL"
  Central axle/2(Central_axle_trq) -> Transfer Case/3
  Central axle/1(Prop_shaft_trq) -> Rear Axle/1(Prop_shaft_trq)
  Veh/1 -> Front Axle/2(Veh), Rear Axle/2(Veh)
  Front Axle/3(Trq_FR) -> Mux/2  "T_FR"
  Rear Axle/3(Tosional_rear_c) -> Central axle/2(Tosional_rear_c)
  Transfer Case/3 -> omega_to_freq_central/1, Front Axle/1(AxlSpd)  "Front axle"
  Transfer Case/4 -> [Axl_centre_Spd], Central axle/1(Rear_axle_speed)  "Centre Axle"
  Front Axle/1(Split torsional Compliance Trq) -> Transfer Case/2
  Front Axle/2(Trq_FL) -> Mux/1  "T_FL"
  Rear Axle/2(Trq_RR) -> Mux/4  "T_RR"
  Transfer Case/1 -> Terminator1/1
  omega_to_freq_central/1 -> Goto/1  "Front_axle_freq"
